simulink library "DoorRlsDriver"  (R2022a)
settings: Solver=VariableStepAuto  StartTime=0.0  StopTime=10.0  RelTol=1e-3
settings Model: Creator=DELL  LastModifiedBy=DELL

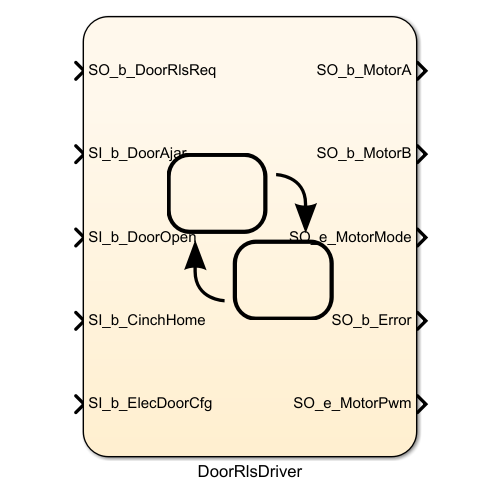
[thumbnail: Simulink's stored preview of the top-level diagram]
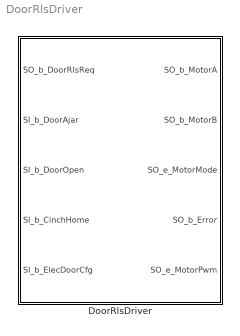
== system DoorRlsDriver ==
  DoorRlsDriver : Stateflow chart  TreatAsAtomicUnit=on

== stateflow chart DoorRlsDriver/DoorRlsDriver ==
  state STARTUP_SETTING
    en:
    SO_b_MotorA=0;
    SO_b_MotorB=1;
    SO_e_MotorMode=2;
    SO_e_MotorPwm=100;
  state NORMAL
    state ELECTRIC_DOOR
      state MAIN_PROGRESS [parallel]
        settings: executionOrder=1
        state RELEASE
          en:
          SL_e_CheckCycle=0;
          SO_e_MotorPwm=100;
          state STEP2_OPEN
            state IDLE
              en:
              SO_b_MotorA=0;
              SO_b_MotorB=0;
              SO_e_MotorMode=0;
            state ERROR
              en:
              SO_b_Error=1;
            state LAST_CHECK
            state ICE_BREAK
            state ERROR1
              en:
              SO_b_Error=1;
            (default) -> NORMAL.ELECTRIC_DOOR.MAIN_PROGRESS.RELEASE.STEP2_OPEN.IDLE
            NORMAL.ELECTRIC_DOOR.MAIN_PROGRESS.RELEASE.STEP2_OPEN.IDLE -> (junction 227) [order 1] : [before(270,tick)&&...
                | SI_b_DoorOpen==0]
            (junction 227) -> (junction 219)
            NORMAL.ELECTRIC_DOOR.MAIN_PROGRESS.RELEASE.STEP2_OPEN.IDLE -> NORMAL.ELECTRIC_DOOR.MAIN_PROGRESS.RELEASE.STEP2_OPEN.LAST_CHECK [order 2] : [after(300,tick)]
            ERROR -> (junction 219)
            NORMAL.ELECTRIC_DOOR.MAIN_PROGRESS.RELEASE.STEP2_OPEN.LAST_CHECK -> ERROR [order 1] : [SI_b_CinchHome!=1]
            (junction 219) -> (junction 210)
            NORMAL.ELECTRIC_DOOR.MAIN_PROGRESS.RELEASE.STEP2_OPEN.LAST_CHECK -> ICE_BREAK [order 2] : [SI_b_CinchHome==1]
            ICE_BREAK -> ERROR1 [order 2] : [after(600,tick)&&...
                | SI_b_CinchHome==1]
            ERROR1 -> (junction 210)
            (junction 210) -> (junction 225)
            ICE_BREAK -> (junction 225) [order 1] : [before(600,tick)&&...
                | hasChangedTo(SI_b_CinchHome,0)]
          state INITIAL
            en:
            SO_b_MotorA=1;
            SO_b_MotorB=0;
            SO_e_MotorMode=1;
            //MotorA=Release Side
          state CHECKING
            en:
            SO_b_MotorA=0;
            SO_b_MotorB=0;
            SO_e_MotorMode=0;
            SL_e_CheckCycle++;
          state RESET
            en:
            SO_b_MotorA=0;
            SO_b_MotorB=1;
            SO_e_MotorMode=2;
            SO_e_MotorPwm=70;
          (default) -> NORMAL.ELECTRIC_DOOR.MAIN_PROGRESS.RELEASE.INITIAL
          NORMAL.ELECTRIC_DOOR.MAIN_PROGRESS.RELEASE.INITIAL -> NORMAL.ELECTRIC_DOOR.MAIN_PROGRESS.RELEASE.CHECKING : [after(30,tick)]
          NORMAL.ELECTRIC_DOOR.MAIN_PROGRESS.RELEASE.CHECKING -> NORMAL.ELECTRIC_DOOR.MAIN_PROGRESS.RELEASE.INITIAL [order 2] : [after(5,tick)&&...
              | SI_b_DoorAjar!=0&&...
              | SL_e_CheckCycle<2]
              | {SO_e_MotorPwm=80;}
          NORMAL.ELECTRIC_DOOR.MAIN_PROGRESS.RELEASE.CHECKING -> NORMAL.ELECTRIC_DOOR.MAIN_PROGRESS.RELEASE.STEP2_OPEN [order 1] : [after(5,tick)&&...
              | SI_b_DoorAjar==0]
          NORMAL.ELECTRIC_DOOR.MAIN_PROGRESS.RELEASE.CHECKING -> NORMAL.ELECTRIC_DOOR.MAIN_PROGRESS.RELEASE.RESET [order 3] : [after(5,tick)&&...
              | SI_b_DoorAjar!=0&&...
              | SL_e_CheckCycle>=2]
          (junction 225) -> NORMAL.ELECTRIC_DOOR.MAIN_PROGRESS.RELEASE.RESET
        state IDLE
          en:
          SO_b_MotorA=0;
          SO_b_MotorB=0;
          SO_e_MotorMode=0;
          SO_e_MotorPwm=0;
          SO_b_Error=0;
        (default) -> NORMAL.ELECTRIC_DOOR.MAIN_PROGRESS.IDLE
        NORMAL.ELECTRIC_DOOR.MAIN_PROGRESS.IDLE -> NORMAL.ELECTRIC_DOOR.MAIN_PROGRESS.RELEASE : [hasChangedTo(SO_b_DoorRlsReq,1)]
        NORMAL.ELECTRIC_DOOR.MAIN_PROGRESS.RELEASE.RESET -> NORMAL.ELECTRIC_DOOR.MAIN_PROGRESS.IDLE : [after(30,tick)]
    state NON_ELECTRIC_DOOR
      state MAIN_PROGRESS [parallel]
        settings: executionOrder=1
        state RELEASE
          en:
          SL_e_CheckCycle=0;
          SO_e_MotorPwm=100;
          state INITIAL
            en:
            SO_b_MotorA=1;
            SO_b_MotorB=0;
            SO_e_MotorMode=1;
            //MotorA=Release Side
          state CHECKING
            en:
            SO_b_MotorA=0;
            SO_b_MotorB=0;
            SO_e_MotorMode=0;
            SL_e_CheckCycle++;
          state STEP2_OPEN
            state IDLE
              en:
              SO_b_MotorA=0;
              SO_b_MotorB=0;
              SO_e_MotorMode=0;
            state LAST_CHECK
            (default) -> NORMAL.NON_ELECTRIC_DOOR.MAIN_PROGRESS.RELEASE.STEP2_OPEN.IDLE
            NORMAL.NON_ELECTRIC_DOOR.MAIN_PROGRESS.RELEASE.STEP2_OPEN.IDLE -> (junction 251) [order 1] : [before(270,tick)&&...
                | SI_b_DoorOpen==0]
            (junction 251) -> (junction 242)
            NORMAL.NON_ELECTRIC_DOOR.MAIN_PROGRESS.RELEASE.STEP2_OPEN.IDLE -> NORMAL.NON_ELECTRIC_DOOR.MAIN_PROGRESS.RELEASE.STEP2_OPEN.LAST_CHECK [order 2] : [after(300,tick)]
            NORMAL.NON_ELECTRIC_DOOR.MAIN_PROGRESS.RELEASE.STEP2_OPEN.LAST_CHECK -> (junction 242)
          state RESET
            en:
            SO_b_MotorA=0;
            SO_b_MotorB=1;
            SO_e_MotorMode=2;
            SO_e_MotorPwm=70;
          (default) -> NORMAL.NON_ELECTRIC_DOOR.MAIN_PROGRESS.RELEASE.INITIAL
          NORMAL.NON_ELECTRIC_DOOR.MAIN_PROGRESS.RELEASE.INITIAL -> NORMAL.NON_ELECTRIC_DOOR.MAIN_PROGRESS.RELEASE.CHECKING : [after(30,tick)]
          NORMAL.NON_ELECTRIC_DOOR.MAIN_PROGRESS.RELEASE.CHECKING -> NORMAL.NON_ELECTRIC_DOOR.MAIN_PROGRESS.RELEASE.STEP2_OPEN [order 1] : [after(5,tick)&&...
              | SI_b_DoorAjar==0]
          NORMAL.NON_ELECTRIC_DOOR.MAIN_PROGRESS.RELEASE.CHECKING -> NORMAL.NON_ELECTRIC_DOOR.MAIN_PROGRESS.RELEASE.INITIAL [order 2] : [after(5,tick)&&...
              | SI_b_DoorAjar!=0&&...
              | SL_e_CheckCycle<2]
              | {SO_e_MotorPwm=80;}
          NORMAL.NON_ELECTRIC_DOOR.MAIN_PROGRESS.RELEASE.CHECKING -> NORMAL.NON_ELECTRIC_DOOR.MAIN_PROGRESS.RELEASE.RESET [order 3] : [after(5,tick)&&...
              | SI_b_DoorAjar!=0&&...
              | SL_e_CheckCycle>=2]
          (junction 242) -> NORMAL.NON_ELECTRIC_DOOR.MAIN_PROGRESS.RELEASE.RESET
        state IDLE
          en:
          SO_b_MotorA=0;
          SO_b_MotorB=0;
          SO_e_MotorMode=0;
          SO_e_MotorPwm=0;
        (default) -> NORMAL.NON_ELECTRIC_DOOR.MAIN_PROGRESS.IDLE
        NORMAL.NON_ELECTRIC_DOOR.MAIN_PROGRESS.IDLE -> NORMAL.NON_ELECTRIC_DOOR.MAIN_PROGRESS.RELEASE : [hasChangedTo(SO_b_DoorRlsReq,1)]
        NORMAL.NON_ELECTRIC_DOOR.MAIN_PROGRESS.RELEASE.RESET -> NORMAL.NON_ELECTRIC_DOOR.MAIN_PROGRESS.IDLE : [after(30,tick)]
    (default) -> ELECTRIC_DOOR [order 1] : [SI_b_ElecDoorCfg]
    (default) -> NON_ELECTRIC_DOOR [order 2]
  (default) -> STARTUP_SETTING
  STARTUP_SETTING -> NORMAL : [after(30,tick)]
  data: SO_b_MotorA output boolean; SO_b_DoorRlsReq input boolean; SI_b_DoorAjar input boolean; SI_b_DoorOpen input boolean; SO_b_MotorB output boolean; SO_e_MotorMode output uint8; SI_b_CinchHome input boolean; SO_b_Error output boolean; SI_b_ElecDoorCfg input boolean; SL_e_CheckCycle local uint8; SO_e_MotorPwm output uint8
